simulink subsystem "celcius_to_fahrenheit_subsystem"  (R2020b)
settings: Solver=VariableStepAuto  StartTime=0.0  StopTime=10.0  RelTol=1e-3
settings Model: Creator=Milind  LastModifiedBy=Milind

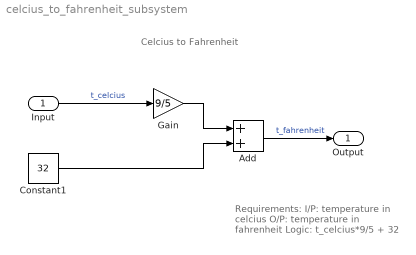
== system celcius_to_fahrenheit_subsystem ==
  note: Requirements:
      | I/P: temperature in celcius
      | O/P: temperature in fahrenheit
      | Logic: t_celcius*9/5 + 32
  note: Celcius to Fahrenheit
  Input : Inport
  Add : Sum
  Constant1 : Constant  Value=32
  Gain : Gain  Gain=9/5
  Output : Outport
  wires:
  Add/1 -> Output/1  "t_fahrenheit"
  Gain/1 -> Add/1
  Constant1/1 -> Add/2
  Input/1 -> Gain/1  "t_celcius"
